simulink model "sldemo_mdlref_outdoor_temp"  (Simulink 7.6)
settings: Solver=ode3  SolverMode=SingleTasking  StartTime=0.0  StopTime=2*24*60*60  FixedStep=60  RelTol=1e-3  AbsTol=1e-6
settings Model: Creator=The MathWorks Inc.  ExtModeAutoUpdateStatusClock=off
settings DataIOCC: ExternalInput=[]  InitialState=[]  LimitDataPoints=off  SaveOutput=off  SaveTime=off
settings OptimizationCC: BlockReduction=off  BooleanDataType=off  InlineParams=on  InlineInvariantSignals=on  InitFltsAndDblsToZero=on
settings DebuggingCC: SaveWithParameterizedLinksMsg=none  CheckExecutionContextPreStartOutputMsg=on  CheckExecutionContextRuntimeOutputMsg=on  SolverPrmCheckMsg=none  MultiTaskDSMMsg=warning  MultiTaskCondExecSysMsg=none  SigSpecEnsureSampleTimeMsg=none  IntegerOverflowMsg=none
settings RTWCC: IncludeERTFirstTime=on
settings CodeAppCC: MaxIdLength=100
settings GRTTargetCC: TargetFcnLib=ansi_tfl_tmw.mat

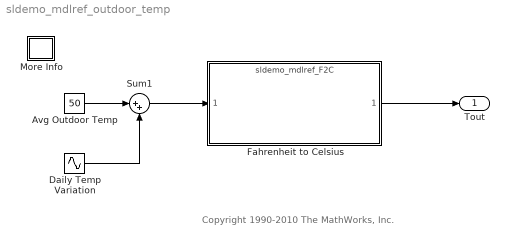
== system sldemo_mdlref_outdoor_temp ==
  note: Copyright 1990-2010 The MathWorks, Inc.
  Avg Outdoor Temp : Constant  Value=50
  Daily Temp Variation : Sin  Amplitude=15  Frequency=2*pi/(24*3600)  SampleTime=0
  Fahrenheit to Celsius : ModelReference  ModelNameDialog=sldemo_mdlref_F2C  SimulationMode=Accelerator  ModelReferenceVersion=1.15  CopyOfModelName=sldemo_mdlref_F2C
  More Info : Subsystem
      settings: OpenFcn=showdemo('sldemo_mdlref_depgraph')
      mask Display: disp('?')
  Sum1 : Sum  Inputs=|++  SaturateOnIntegerOverflow=on  InputSameDT=on  OutDataTypeStr=Inherit: Same as first input
  Tout : Outport
  wires:
  Fahrenheit to Celsius/1 -> Tout/1
  Avg Outdoor Temp/1 -> Sum1/1
  Sum1/1 -> Fahrenheit to Celsius/1
  Daily Temp Variation/1 -> Sum1/2

== system sldemo_mdlref_outdoor_temp/More Info ==
